simulink model "Arch_Plotter_System"  (R2024b)
settings: Solver=VariableStepAuto  StartTime=0.0  StopTime=10.0  RelTol=1e-3
settings Model: Creator=Niels  LastModifiedBy=Niels

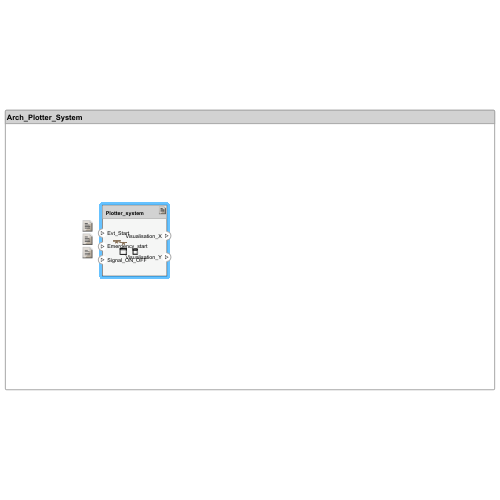
[thumbnail: Simulink's stored preview of the top-level diagram]
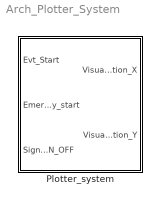
== system Arch_Plotter_System ==
  Plotter_system : Subsystem
      settings: PortSchema="{\"entries\":[{\"content\":{\"headerSize\":26,\"margin\":15,\"minimumSpacing\":25,\"sides\":[{\"content\":{\"connectorIds\":[\"In1\",\"In2\",\"In3\"]},\"type\":\"ConnectorPlacement.EquallySpacedRectSide\",\"uuid\":\"77cc6d80-45a7-42c2-8352-1aa42436139f\"},{\"content\":{\"connectorIds\":[\"Out1\",\"Out2\"],\"side\":\"RIGHT\"},\"type\":\"ConnectorPlacement.EquallySpacedRectSide\",\"uuid\":\"fb2d4574-b331-450e-9bfa-0e573c015a2c\"},{\"content\":{\"side\":\"TOP\"},\"type\":\"ConnectorPlacement.EquallySpacedRectSide\",\"uuid\":\"8af6ec5c-e17c-482b-ba32-4684d975b613\"}]},\"type\":\"ConnectorPlacement.EquallySpacedConnector\",\"uuid\":\"eaa89c3b-b5bf-4a4b-98ff-a7b3b5e85f4e\"}],\"packageUris\":[\"http://schema.mathworks.com/mf0/Connector/R2020b\"],\"version\":\"1.0\"}"

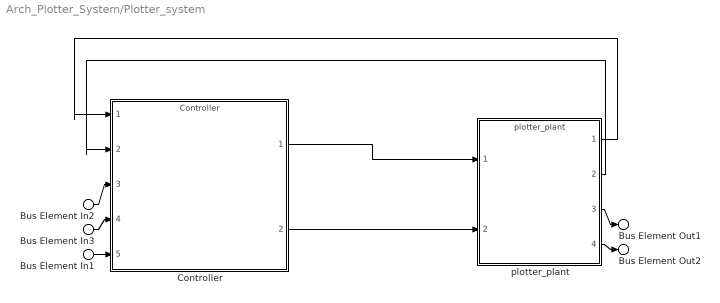
== system Arch_Plotter_System/Plotter_system ==
  Bus Element In2 : Inport  PortName=Evt_Start
  Bus Element In3 : Inport  Port=2  PortName=Emergency_start
  Bus Element In1 : Inport  Port=3  PortName=Signal_ON_OFF
  Controller : ModelReference  ModelNameDialog=Controller  SimulationMode=Normal  ModelReferenceVersion=1.1
      settings: PortSchema="{\"entries\":[{\"content\":{\"headerSize\":38,\"margin\":15,\"minimumSpacing\":25,\"sides\":[{\"content\":{\"connectorIds\":[\"In1\",\"In2\",\"In3\",\"In4\",\"In5\"]},\"type\":\"ConnectorPlacement.EquallySpacedRectSide\",\"uuid\":\"77cc6d80-45a7-42c2-8352-1aa42436139f\"},{\"content\":{\"connectorIds\":[\"Out1\",\"Out2\"],\"side\":\"RIGHT\"},\"type\":\"ConnectorPlacement.EquallySpacedRectSide\",\"uuid\":\"fb2d4574-b331-450e-9bfa-0e573c015a2c\"},{\"content\":{\"side\":\"TOP\"},\"type\":\"ConnectorPlacement.EquallySpacedRectSide\",\"uuid\":\"8af6ec5c-e17c-482b-ba32-4684d975b613\"}]},\"type\":\"ConnectorPlacement.EquallySpacedConnector\",\"uuid\":\"eaa89c3b-b5bf-4a4b-98ff-a7b3b5e85f4e\"}],\"packageUris\":[\"http://schema.mathworks.com/mf0/Connector/R2020b\"],\"version\":\"1.0\"}"
  plotter_plant : ModelReference  ModelNameDialog=plotter_plant  SimulationMode=Normal  ModelReferenceVersion=1.3
      settings: PortSchema="{\"entries\":[{\"content\":{\"headerSize\":38,\"margin\":15,\"minimumSpacing\":25,\"sides\":[{\"content\":{\"connectorIds\":[\"In1\",\"In2\"]},\"type\":\"ConnectorPlacement.EquallySpacedRectSide\",\"uuid\":\"77cc6d80-45a7-42c2-8352-1aa42436139f\"},{\"content\":{\"connectorIds\":[\"Out1\",\"Out2\",\"Out3\",\"Out4\"],\"side\":\"RIGHT\"},\"type\":\"ConnectorPlacement.EquallySpacedRectSide\",\"uuid\":\"fb2d4574-b331-450e-9bfa-0e573c015a2c\"},{\"content\":{\"side\":\"TOP\"},\"type\":\"ConnectorPlacement.EquallySpacedRectSide\",\"uuid\":\"8af6ec5c-e17c-482b-ba32-4684d975b613\"}]},\"type\":\"ConnectorPlacement.EquallySpacedConnector\",\"uuid\":\"eaa89c3b-b5bf-4a4b-98ff-a7b3b5e85f4e\"}],\"packageUris\":[\"http://schema.mathworks.com/mf0/Connector/R2020b\"],\"version\":\"1.0\"}"
  Bus Element Out2 : Outport  PortName=Visualisation_X
  Bus Element Out1 : Outport  Port=2  PortName=Visualisation_Y
  wires:
  plotter_plant/4 -> Bus Element Out2/1
  plotter_plant/3 -> Bus Element Out1/1
  Bus Element In3/1 -> Controller/4
  Bus Element In2/1 -> Controller/3
  Bus Element In1/1 -> Controller/5
  plotter_plant/1 -> Controller/1
  plotter_plant/2 -> Controller/2
  Controller/2 -> plotter_plant/2
  Controller/1 -> plotter_plant/1
